simulink model "Stirred_tank_heater_Fuzzy_Control"  (R2017b)
settings: Solver=VariableStepAuto  StartTime=0.0  StopTime=4  RelTol=1e-3
libraries: fuzblock x1
settings Model: Creator=HP  LastModifiedBy=HP

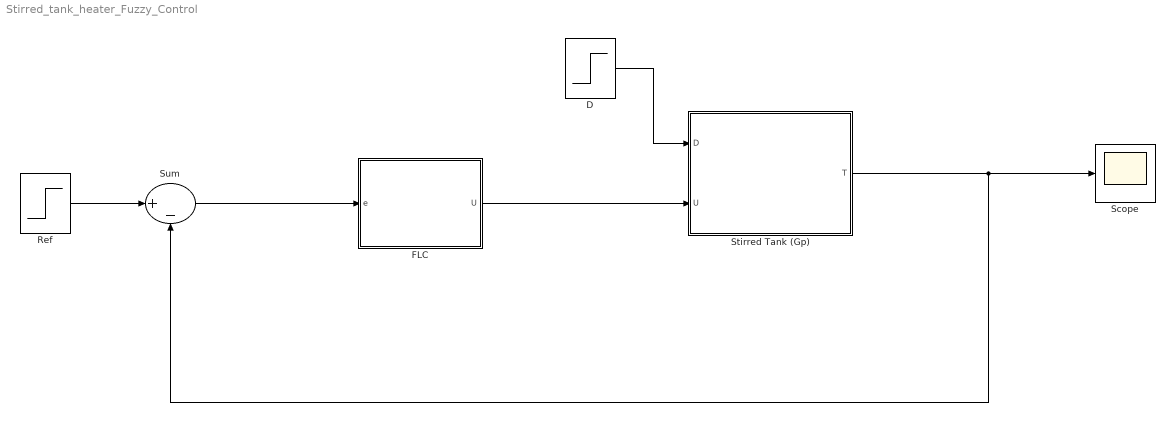
== system Stirred_tank_heater_Fuzzy_Control ==
  D : Step  Time=2  After=0  SampleTime=0.01
  FLC : Subsystem
  Ref : Step  Time=0  SampleTime=0.01
  Scope : Scope
  Stirred Tank (Gp) : Subsystem
  Sum : Sum  Inputs=|+-
  wires:
  Stirred Tank (Gp)/1(T) -> Scope/1, Sum/2
  Ref/1 -> Sum/1
  D/1 -> Stirred Tank (Gp)/1(D)
  FLC/1(U) -> Stirred Tank (Gp)/2(U)
  Sum/1 -> FLC/1(e)

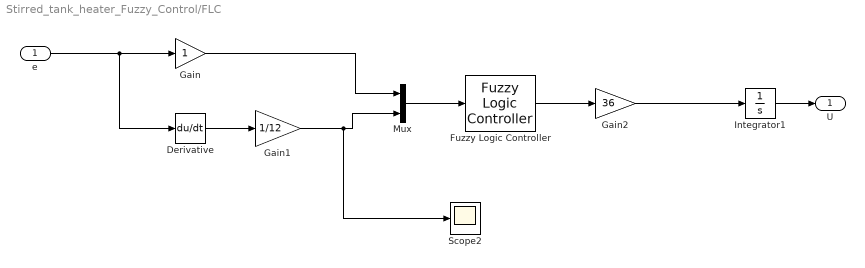
== system Stirred_tank_heater_Fuzzy_Control/FLC ==
  e : Inport
  Derivative : Derivative
  Fuzzy Logic Controller : fuzblock/Fuzzy Logic  Controller  FIS='Stirred_Tank_Temp_PIFLC'  OutputSampleNumber=101  DataType=double  FuzzifiedInputs=off  RuleFiringStrengths=off  RuleOutputs=off  AggregatedOutputs=off  SimulateUsing=Interpreted execution
  Gain : Gain
  Gain1 : Gain  Gain=1/12
  Gain2 : Gain  Gain=36
  Integrator1 : Integrator
  Mux : Mux  Inputs=2
  Scope2 : Scope
  U : Outport
  wires:
  e/1 -> Gain/1, Derivative/1
  Gain/1 -> Mux/1
  Derivative/1 -> Gain1/1
  Gain1/1 -> Mux/2, Scope2/1
  Mux/1 -> Fuzzy Logic Controller/1
  Fuzzy Logic Controller/1 -> Gain2/1
  Gain2/1 -> Integrator1/1
  Integrator1/1 -> U/1

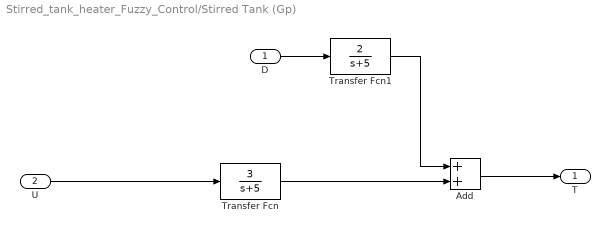
== system Stirred_tank_heater_Fuzzy_Control/Stirred Tank (Gp) ==
  D : Inport
  U : Inport  Port=2
  Add : Sum
  Transfer Fcn : TransferFcn  Numerator=[3]  Denominator=[1 5]
  Transfer Fcn1 : TransferFcn  Numerator=[2]  Denominator=[1 5]
  T : Outport
  wires:
  U/1 -> Transfer Fcn/1
  Add/1 -> T/1
  Transfer Fcn/1 -> Add/2
  Transfer Fcn1/1 -> Add/1
  D/1 -> Transfer Fcn1/1
